simulink subsystem "IF"  (R2024b)
settings: Solver=VariableStepAuto  StartTime=0.0  StopTime=10.0  RelTol=1e-3
values from neighbouring files (symbols this model uses):
  entryPointAddress = hex2dec('80000000')    [initSimuRISC.m]
  instructionMemory = uint32(zeros(2^SimuRISC_Constants.DATATYPE_MEMORY_ADDR.WordLength , 1))    [initSimuRISC.m]
undefined symbols (not defined in the file or in its folder): SimuRISC_Constants
libraries: simulink x9, hdlsllib x1
settings Model: Creator=stefano  LastModifiedBy=stefano

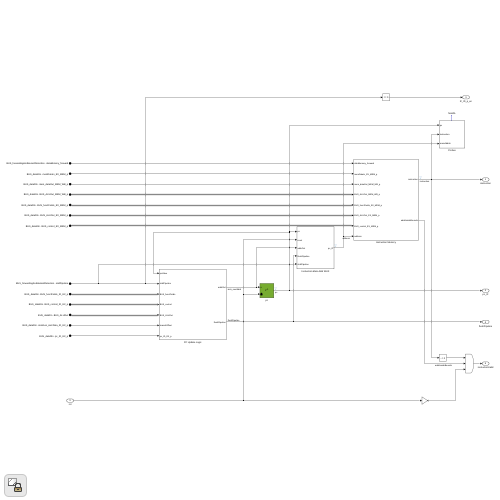
[thumbnail: Simulink's stored preview of the top-level diagram]
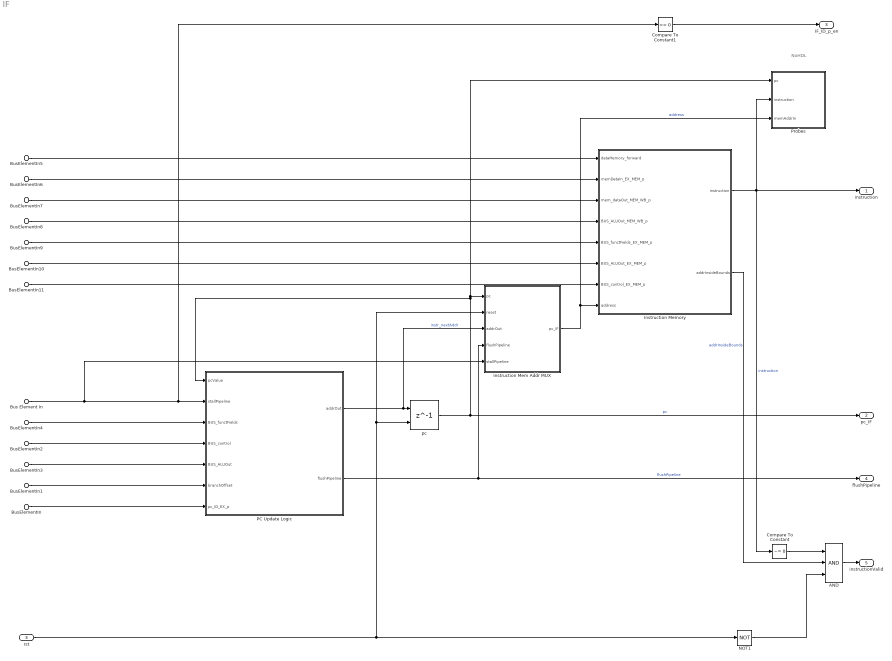
== system IF ==
  note: NoHDL
  BusElementIn : Inport  PortName=BUS_dataRtn  Element=pc_ID_EX_p
  BusElementIn1 : Inport  PortName=BUS_dataRtn  Element=immGen_instrData_ID_EX_p
  BusElementIn2 : Inport  PortName=BUS_dataRtn  Element=BUS_control_ID_EX_p
  BusElementIn3 : Inport  PortName=BUS_dataRtn  Element=BUS_ALUOut
  BusElementIn4 : Inport  PortName=BUS_dataRtn  Element=BUS_functFields_ID_EX_p
  BusElementIn6 : Inport  PortName=BUS_dataRtn  Element=memDataIn_EX_MEM_p
  BusElementIn7 : Inport  PortName=BUS_dataRtn  Element=mem_dataOut_MEM_WB_p
  BusElementIn8 : Inport  PortName=BUS_dataRtn  Element=BUS_ALUOut_MEM_WB_p
  BusElementIn9 : Inport  PortName=BUS_dataRtn  Element=BUS_functFields_EX_MEM_p
  BusElementIn10 : Inport  PortName=BUS_dataRtn  Element=BUS_ALUOut_EX_MEM_p
  BusElementIn11 : Inport  PortName=BUS_dataRtn  Element=BUS_control_EX_MEM_p
  Bus Element In : Inport  Port=2  PortName=BUS_forwardingAndHazardDetection  Element=stallPipeline
  BusElementIn5 : Inport  Port=2  PortName=BUS_forwardingAndHazardDetection  Element=dataMemory_forward
  rst : Inport  Port=3
  AND : Logic  Inputs=3  IconShape=distinctive  AllPortsSameDT=off  OutDataTypeStr=boolean
  Compare To Constant : simulink/Logic and Bit Operations/Compare To Constant  relop=~=  const=0  OutDataTypeStr=boolean
  Compare To Constant1 : simulink/Logic and Bit Operations/Compare To Constant  relop===  const=0  OutDataTypeStr=boolean
  Instruction Mem Addr MUX : Subsystem
  Instruction Memory : Subsystem
  NOT1 : Logic  Operator=NOT  IconShape=distinctive  AllPortsSameDT=off  OutDataTypeStr=boolean
  PC Update Logic : Subsystem
  Probes : Subsystem
  pc : Delay  DelayLength=1  InitialCondition=entryPointAddress  ExternalReset=Level hold
      settings: InputPortMap=u0,r5
  instruction : Outport
  pc_IF : Outport  Port=2
  IF_ID_p_en : Outport  Port=3
  flushPipeline : Outport  Port=4
  instructionValid : Outport  Port=5
  wires:
  PC Update Logic/2(flushPipeline) -> Instruction Mem Addr MUX/4(flushPipeline), flushPipeline/1  "flushPipeline"
  Instruction Memory/1(instruction) -> Probes/2(instruction), instruction/1, Compare To Constant/1  "instruction"
  BusElementIn3/1 -> PC Update Logic/5(BUS_ALUOut)
  BusElementIn2/1 -> PC Update Logic/4(BUS_control)
  rst/1 -> NOT1/1, pc/2, Instruction Mem Addr MUX/2(reset)
  BusElementIn1/1 -> PC Update Logic/6(branchOffset)
  BusElementIn/1 -> PC Update Logic/7(pc_ID_EX_p)
  BusElementIn4/1 -> PC Update Logic/3(BUS_functFields)
  pc/1 -> PC Update Logic/1(pcValue), Instruction Mem Addr MUX/1(pc), Probes/1(pc), pc_IF/1  "pc"
  Bus Element In/1 -> PC Update Logic/2(stallPipeline), Compare To Constant1/1, Instruction Mem Addr MUX/5(stallPipeline)
  PC Update Logic/1(addrOut) -> pc/1, Instruction Mem Addr MUX/3(addrOut)  "instr_nextAddr"
  AND/1 -> instructionValid/1
  Instruction Memory/2(addrInsideBounds) -> AND/2  "addrInsideBounds"
  NOT1/1 -> AND/3
  Compare To Constant/1 -> AND/1
  BusElementIn5/1 -> Instruction Memory/1(dataMemory_forward)
  BusElementIn7/1 -> Instruction Memory/3(mem_dataOut_MEM_WB_p)
  BusElementIn8/1 -> Instruction Memory/4(BUS_ALUOut_MEM_WB_p)
  BusElementIn6/1 -> Instruction Memory/2(memDataIn_EX_MEM_p)
  BusElementIn9/1 -> Instruction Memory/5(BUS_functFields_EX_MEM_p)
  BusElementIn10/1 -> Instruction Memory/6(BUS_ALUOut_EX_MEM_p)
  BusElementIn11/1 -> Instruction Memory/7(BUS_control_EX_MEM_p)
  Instruction Mem Addr MUX/1(pc_IF) -> Instruction Memory/8(address), Probes/3(memAddrIn)  "address"
  Compare To Constant1/1 -> IF_ID_p_en/1

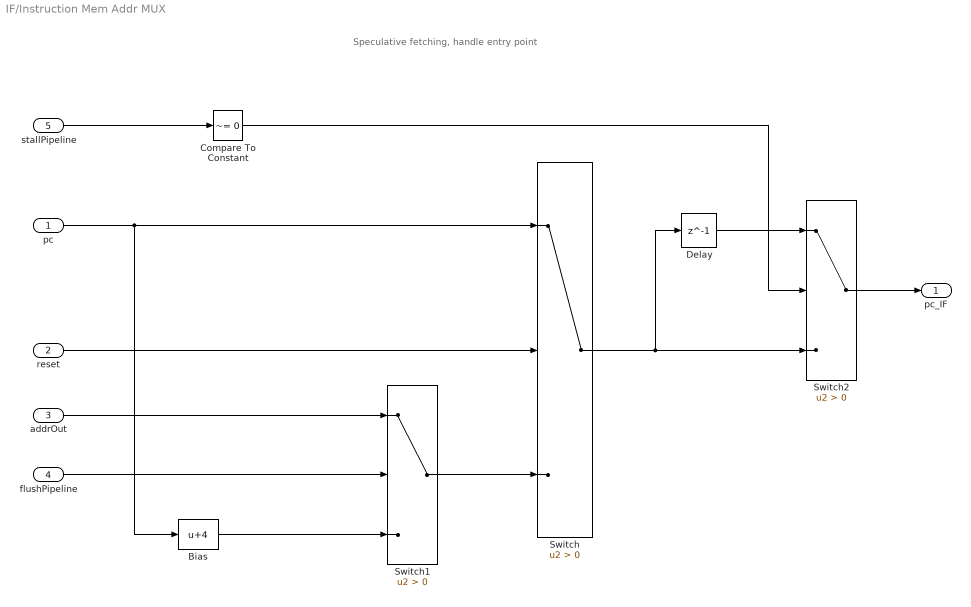
== system IF/Instruction Mem Addr MUX ==
  note: Speculative fetching, handle entry point
  pc : Inport
  reset : Inport  Port=2
  addrOut : Inport  Port=3
  flushPipeline : Inport  Port=4
  stallPipeline : Inport  Port=5
  Bias : Bias  Bias=4  SaturateOnIntegerOverflow=off
  Compare To Constant : simulink/Logic and Bit Operations/Compare To Constant  relop=~=  const=0  OutDataTypeStr=boolean
  Delay : Delay  DelayLength=1
  Switch : Switch  Criteria=u2 > Threshold  SaturateOnIntegerOverflow=off  InputSameDT=off
  Switch1 : Switch  Criteria=u2 > Threshold  SaturateOnIntegerOverflow=off  InputSameDT=off
  Switch2 : Switch  Criteria=u2 > Threshold  SaturateOnIntegerOverflow=off  InputSameDT=off
  pc_IF : Outport
  wires:
  Delay/1 -> Switch2/1
  Switch/1 -> Switch2/3, Delay/1
  Compare To Constant/1 -> Switch2/2
  stallPipeline/1 -> Compare To Constant/1
  addrOut/1 -> Switch1/1
  flushPipeline/1 -> Switch1/2
  Switch1/1 -> Switch/3
  Bias/1 -> Switch1/3
  pc/1 -> Switch/1, Bias/1
  reset/1 -> Switch/2
  Switch2/1 -> pc_IF/1

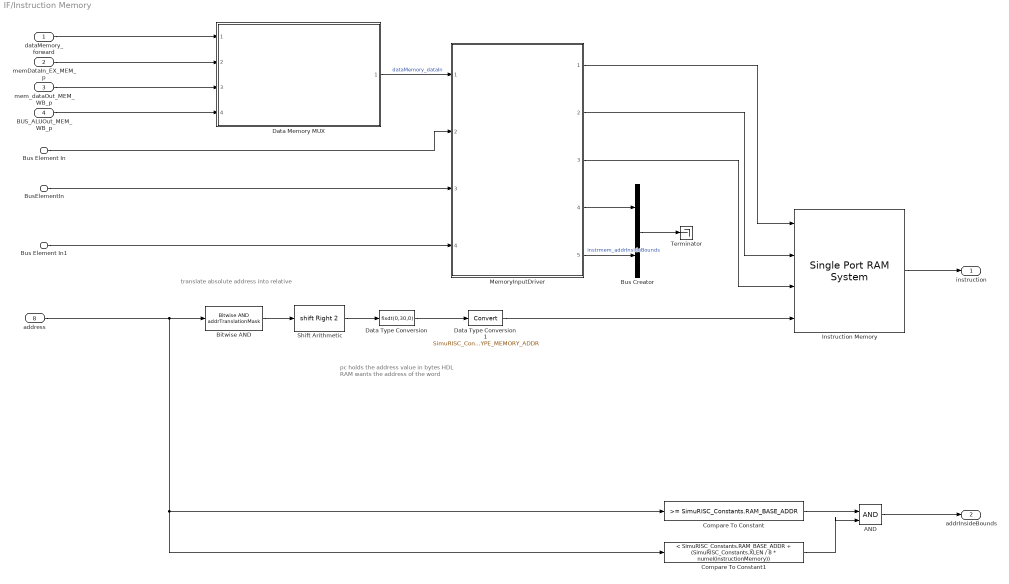
== system IF/Instruction Memory ==
  note: pc holds the address value in bytes
      | HDL RAM wants the address of the word
  note: translate absolute address into relative
  dataMemory_forward : Inport
  memDataIn_EX_MEM_p : Inport  Port=2
  mem_dataOut_MEM_WB_p : Inport  Port=3
  BUS_ALUOut_MEM_WB_p : Inport  Port=4
  Bus Element In : Inport  Port=5  PortName=BUS_functFields_EX_MEM_p  Element=funct3
  Bus Element In1 : Inport  Port=6  PortName=BUS_ALUOut_EX_MEM_p  Element=result
  BusElementIn : Inport  Port=7  PortName=BUS_control_EX_MEM_p  Element=memWrite
  address : Inport  Port=8
  AND : Logic  IconShape=distinctive  AllPortsSameDT=off  OutDataTypeStr=boolean
  Bitwise AND : simulink/Logic and Bit Operations/Bitwise Operator  logicop=AND  UseBitMask=on  BitMask=addrTranslationMask  BitMaskRealWorld=Stored Integer
      settings: LibrarySourceBlock=|
      | simulink/Quick Insert/Logic and Bit
      | Operations/Bitwise AND
  Bus Creator : BusCreator  Inputs=2
  Compare To Constant : simulink/Logic and Bit Operations/Compare To Constant  relop=>=  const=SimuRISC_Constants.RAM_BASE_ADDR  OutDataTypeStr=boolean
  Compare To Constant1 : simulink/Logic and Bit Operations/Compare To Constant  relop=<  const=SimuRISC_Constants.RAM_BASE_ADDR + (SimuRISC_Constants.XLEN / 8 * numel(instructionMemory))  OutDataTypeStr=boolean
  Data Memory MUX : Subsystem  ReferencedSubsystem=DataMemoryMUX
  Data Type Conversion : DataTypeConversion  OutDataTypeStr=fixdt(0,30,0)  SaturateOnIntegerOverflow=off  RndMeth=Floor
  Data Type Conversion1 : DataTypeConversion  OutDataTypeStr=SimuRISC_Constants.DATATYPE_MEMORY_ADDR  SaturateOnIntegerOverflow=off  RndMeth=Floor
  Instruction Memory : hdlsllib/HDL RAMs/Single Port RAM System  RAMType=Simple dual port  AsyncRead=off  WriteOutputValue=New data  RAMInitialValue=instructionMemory  allowBusInputs=off  WritesHaveOutput=on  NumReads=0  NumWrites=1  SimulateUsing=Code generation  ModelRAMDelay=on
  MemoryInputDriver : Subsystem  ReferencedSubsystem=MemoryInputDriver  absoluteAddress=SimuRISC_Constants.RAM_BASE_ADDR  MemoryNWords=numel(instructionMemory)  registerDataType=registerDataType
  Shift Arithmetic : ArithShift  BitShiftNumber=2  BitShiftDirection=Right
  Terminator : Terminator
  instruction : Outport
  addrInsideBounds : Outport  Port=2
  wires:
  AND/1 -> addrInsideBounds/1
  Compare To Constant/1 -> AND/1
  Compare To Constant1/1 -> AND/2
  Bus Creator/1 -> Terminator/1
  MemoryInputDriver/5 -> Bus Creator/2  "instrmem_addrInsideBounds"
  MemoryInputDriver/4 -> Bus Creator/1
  MemoryInputDriver/3 -> Instruction Memory/3
  MemoryInputDriver/2 -> Instruction Memory/2
  MemoryInputDriver/1 -> Instruction Memory/1
  BusElementIn/1 -> MemoryInputDriver/3
  Bus Element In1/1 -> MemoryInputDriver/4
  Bus Element In/1 -> MemoryInputDriver/2
  Data Memory MUX/1 -> MemoryInputDriver/1  "dataMemory_dataIn"
  BUS_ALUOut_MEM_WB_p/1 -> Data Memory MUX/4
  mem_dataOut_MEM_WB_p/1 -> Data Memory MUX/3
  memDataIn_EX_MEM_p/1 -> Data Memory MUX/2
  dataMemory_forward/1 -> Data Memory MUX/1
  Bitwise AND/1 -> Shift Arithmetic/1
  address/1 -> Bitwise AND/1, Compare To Constant/1, Compare To Constant1/1
  Data Type Conversion/1 -> Data Type Conversion1/1
  Shift Arithmetic/1 -> Data Type Conversion/1
  Instruction Memory/1 -> instruction/1
  Data Type Conversion1/1 -> Instruction Memory/4

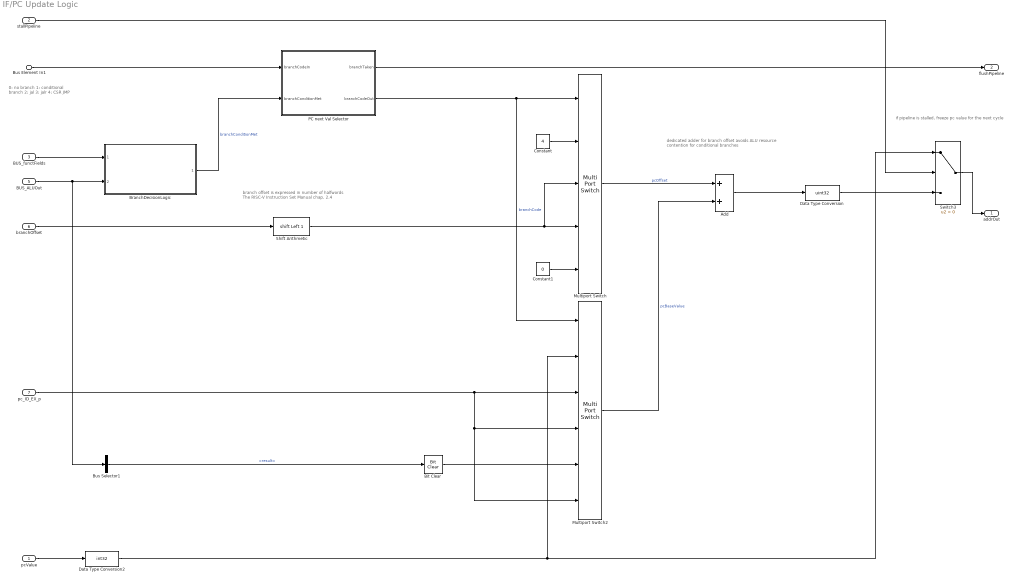
== system IF/PC Update Logic ==
  note: branch offset is expressed in number of halfwords
      | The RISC-V Instruction Set Manual chap. 2.4
  note: dedicated adder for branch offset
      | avoids ALU resource contention for conditional branches
  note: 0: no branch
      | 1: conditional branch
      | 2: jal
      | 3: jalr
      | 4: CSR JMP
  note: if pipeline is stalled, freeze pc value for the next cycle
  pcValue : Inport
  stallPipeline : Inport  Port=2
  BUS_functFields : Inport  Port=3
  Bus Element In1 : Inport  Port=4  PortName=BUS_control  Element=branch
  BUS_ALUOut : Inport  Port=5
  branchOffset : Inport  Port=6
  pc_ID_EX_p : Inport  Port=7
  Add : Sum  OutDataTypeStr=Inherit: Same as first input
  Bit Clear : simulink/Logic and Bit Operations/Bit Clear  iBit=0
  BranchDecisionLogic : Subsystem  ReferencedSubsystem=BranchDecisionLogic
  Bus Selector1 : BusSelector  OutputSignals=result
  Constant : Constant  Value=4  OutDataTypeStr=int32  SampleTime=-1
  Constant1 : Constant  Value=0  OutDataTypeStr=int32  SampleTime=-1
  Data Type Conversion : DataTypeConversion  OutDataTypeStr=uint32  ConvertRealWorld=Stored Integer (SI)  SaturateOnIntegerOverflow=off  RndMeth=Floor
  Data Type Conversion2 : DataTypeConversion  OutDataTypeStr=int32  ConvertRealWorld=Stored Integer (SI)  SaturateOnIntegerOverflow=off  RndMeth=Floor
  Multiport Switch : MultiPortSwitch  DataPortOrder=Zero-based contiguous  Inputs=4  DiagnosticForDefault=None  zeroidx=on  SaturateOnIntegerOverflow=off  InputSameDT=off
  Multiport Switch2 : MultiPortSwitch  DataPortOrder=Zero-based contiguous  Inputs=5  DiagnosticForDefault=None  zeroidx=on  SaturateOnIntegerOverflow=off  InputSameDT=off
  PC next Val Selector : Subsystem
  Shift Arithmetic : ArithShift  BitShiftNumber=1  BitShiftDirection=Left
  Switch3 : Switch  Criteria=u2 > Threshold  SaturateOnIntegerOverflow=off  InputSameDT=off
  addrOut : Outport
  flushPipeline : Outport  Port=2
  wires:
  Data Type Conversion2/1 -> Multiport Switch2/2, Switch3/1
  PC next Val Selector/2(branchCodeOut) -> Multiport Switch/1, Multiport Switch2/1  "branchCode"
  PC next Val Selector/1(branchTaken) -> flushPipeline/1
  Multiport Switch2/1 -> Add/2  "pcBaseValue"
  pc_ID_EX_p/1 -> Multiport Switch2/4, Multiport Switch2/6, Multiport Switch2/3
  pcValue/1 -> Data Type Conversion2/1
  stallPipeline/1 -> Switch3/2
  Switch3/1 -> addrOut/1
  Add/1 -> Data Type Conversion/1
  Bit Clear/1 -> Multiport Switch2/5
  Constant1/1 -> Multiport Switch/5
  Bus Element In1/1 -> PC next Val Selector/1(branchCodeIn)
  Multiport Switch/1 -> Add/1  "pcOffset"
  Bus Selector1/1 -> Bit Clear/1  "<result>"
  Data Type Conversion/1 -> Switch3/3
  branchOffset/1 -> Shift Arithmetic/1
  BUS_ALUOut/1 -> BranchDecisionLogic/2, Bus Selector1/1
  BUS_functFields/1 -> BranchDecisionLogic/1
  BranchDecisionLogic/1 -> PC next Val Selector/2(branchConditionMet)  "branchConditionMet"
  Shift Arithmetic/1 -> Multiport Switch/4, Multiport Switch/3
  Constant/1 -> Multiport Switch/2

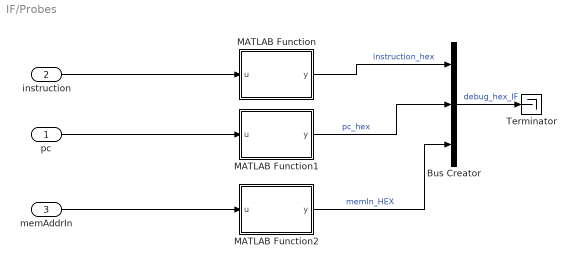
== system IF/Probes ==
  pc : Inport
  instruction : Inport  Port=2
  memAddrIn : Inport  Port=3
  Bus Creator : BusCreator  Inputs=3
  MATLAB Function : MATLAB Function  TreatAsAtomicUnit=on
  MATLAB Function1 : MATLAB Function  TreatAsAtomicUnit=on
  MATLAB Function2 : MATLAB Function  TreatAsAtomicUnit=on
  Terminator : Terminator
  wires:
  memAddrIn/1 -> MATLAB Function2/1(u)
  MATLAB Function2/1(y) -> Bus Creator/3  "memIn_HEX"
  MATLAB Function1/1(y) -> Bus Creator/2  "pc_hex"
  Bus Creator/1 -> Terminator/1  "debug_hex_IF"
  instruction/1 -> MATLAB Function/1(u)
  pc/1 -> MATLAB Function1/1(u)
  MATLAB Function/1(y) -> Bus Creator/1  "instruction_hex"

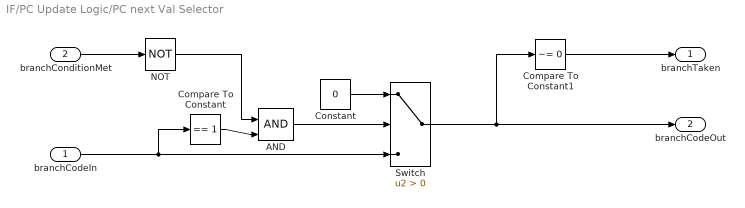
== system IF/PC Update Logic/PC next Val Selector ==
  branchCodeIn : Inport
  branchConditionMet : Inport  Port=2
  AND : Logic  IconShape=distinctive  AllPortsSameDT=off  OutDataTypeStr=boolean
  Compare To Constant : simulink/Logic and Bit Operations/Compare To Constant  relop===  const=1  OutDataTypeStr=boolean
  Compare To Constant1 : simulink/Logic and Bit Operations/Compare To Constant  relop=~=  const=0  OutDataTypeStr=boolean
  Constant : Constant  Value=0  OutDataTypeStr=fixdt(0,3,0)  SampleTime=-1
  NOT : Logic  Operator=NOT  IconShape=distinctive  AllPortsSameDT=off  OutDataTypeStr=boolean
  Switch : Switch  Criteria=u2 > Threshold  SaturateOnIntegerOverflow=off  InputSameDT=off
  branchTaken : Outport
  branchCodeOut : Outport  Port=2
  wires:
  Constant/1 -> Switch/1
  Compare To Constant1/1 -> branchTaken/1
  Switch/1 -> branchCodeOut/1, Compare To Constant1/1
  AND/1 -> Switch/2
  NOT/1 -> AND/1
  Compare To Constant/1 -> AND/2
  branchConditionMet/1 -> NOT/1
  branchCodeIn/1 -> Switch/3, Compare To Constant/1

== matlab function IF/Probes/MATLAB Function1 ==
  data: u input; y output string
function y = toHex(u)

y = string(dec2hex(u, 8));

== matlab function IF/Probes/MATLAB Function2 ==
  data: u input; y output string
function y = toHex(u)

y = string(dec2hex(u, 8));

== matlab function IF/Probes/MATLAB Function ==
  data: u input; y output string
function y = toHex(u)

y = string(dec2hex(u, 8));
